simulink model "liftsubsystem"  (R2025b)
settings: Solver=daessc  StartTime=0.0  StopTime=15  FixedStep=1e-3  RelTol=1e-3
values from neighbouring files (symbols this model uses):
  b0 = 1.0    (= 1)    [get_arm_model_with_disturbance.m]    (also in robotParams.m = 3.125)
  beta1 = 3 * omega_o    (= 120)    [robotParams.m]
  beta2 = 3 * omega_o^2    (= 4800)    [robotParams.m]
  beta3 = omega_o^3    (= 64000)    [robotParams.m]
  g = 9.81    [get_arm_model.m]    (also in robotParams.m)
  g_fork = 2*pi*50    (= 314.159265359)    [robotParams.m]
  g_lift = 2*pi*50    (= 314.159265359)    [robotParams.m]
  Kd_fork = 5    [robotParams.m]
  Kd_lift = 5    [robotParams.m]
  Kp_fork = 20    [robotParams.m]
  Kp_lift = 20    [robotParams.m]
  lx = 0.3    [robotParams.m]
  ly = 0.8    [robotParams.m]
  lz = 1    [robotParams.m]
  m = 1    [robotParams.m]
  M = reshape([mt1,mt2,mt3],4,4)    [mass_matrix.m]    (also in robotParams.m = 16)
  m_w = 1    [robotParams.m]
  N = 20    [ocp_arm.m]    (also in ocp_arm_disturbances.m; ocp_lift.m)
  T_control = 1e-3    (= 0.001)    [robotParams.m]
undefined symbols (not defined in the file or in its folder): dspblkCoreblockFVToolHelper, gcbh, K_fd, K_fp, M_n44, Mn_33, Mn_44, X, Y, Z
libraries: sm_lib x257, nesl_utility x58, sharedTrackingLibrary x6, slpidlib x4, simulink x4, robotcorelib x1
(part 2 of 8)

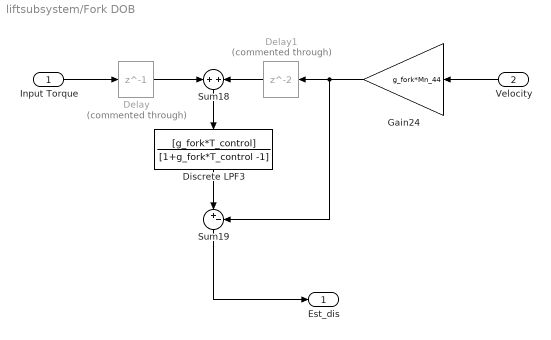
== system liftsubsystem/Fork DOB ==
  Input Torque : Inport
  Velocity : Inport  Port=2
  Delay : Delay  Commented=through  DelayLength=1  InputProcessing=Columns as channels (frame based)  SampleTime=T_control
  Delay1 : Delay  Commented=through  InputProcessing=Columns as channels (frame based)  SampleTime=T_control
  Discrete LPF3 : DiscreteFilter  LoadFcn=dspblkCoreblockFVToolHelper(gcbh,'load');  Numerator=[g_fork*T_control]  Denominator=[1+g_fork*T_control -1]
      settings: CopyFcn=dspblkCoreblockFVToolHelper(gcbh,'copy');  DeleteFcn=dspblkCoreblockFVToolHelper(gcbh,'close');  ModelCloseFcn=dspblkCoreblockFVToolHelper(gcbh,'close');  PreSaveFcn=dspblkCoreblockFVToolHelper(gcbh,'presave');  PostSaveFcn=dspblkCoreblockFVToolHelper(gcbh,'postsave');  CloseFcn=dspblkCoreblockFVToolHelper(gcbh,'close');
  Gain24 : Gain  Gain=g_fork*Mn_44
  Sum18 : Sum  Inputs=+|+
  Sum19 : Sum  Inputs=|+-
  Est_dis : Outport
  wires:
  Delay/1 -> Sum18/1
  Sum19/1 -> Est_dis/1
  Velocity/1 -> Gain24/1
  Input Torque/1 -> Delay/1
  Sum18/1 -> Discrete LPF3/1
  Gain24/1 -> Sum19/2, Delay1/1
  Discrete LPF3/1 -> Sum19/1
  Delay1/1 -> Sum18/2

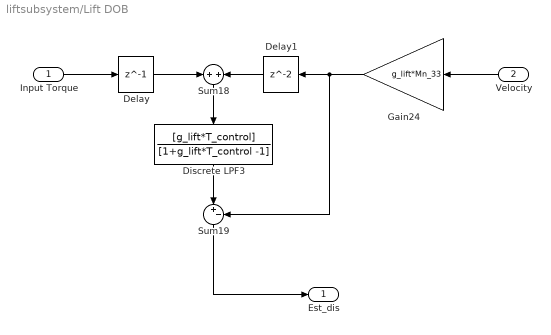
== system liftsubsystem/Lift DOB ==
  Input Torque : Inport
  Velocity : Inport  Port=2
  Delay : Delay  DelayLength=1  InputProcessing=Columns as channels (frame based)  SampleTime=T_control
  Delay1 : Delay  InputProcessing=Columns as channels (frame based)  SampleTime=T_control
  Discrete LPF3 : DiscreteFilter  LoadFcn=dspblkCoreblockFVToolHelper(gcbh,'load');  Numerator=[g_lift*T_control]  Denominator=[1+g_lift*T_control -1]
      settings: CopyFcn=dspblkCoreblockFVToolHelper(gcbh,'copy');  DeleteFcn=dspblkCoreblockFVToolHelper(gcbh,'close');  ModelCloseFcn=dspblkCoreblockFVToolHelper(gcbh,'close');  PreSaveFcn=dspblkCoreblockFVToolHelper(gcbh,'presave');  PostSaveFcn=dspblkCoreblockFVToolHelper(gcbh,'postsave');  CloseFcn=dspblkCoreblockFVToolHelper(gcbh,'close');
  Gain24 : Gain  Gain=g_lift*Mn_33
  Sum18 : Sum  Inputs=+|+
  Sum19 : Sum  Inputs=|+-
  Est_dis : Outport
  wires:
  Delay1/1 -> Sum18/2
  Discrete LPF3/1 -> Sum19/1
  Gain24/1 -> Delay1/1, Sum19/2
  Sum18/1 -> Discrete LPF3/1
  Input Torque/1 -> Delay/1
  Velocity/1 -> Gain24/1
  Sum19/1 -> Est_dis/1
  Delay/1 -> Sum18/1

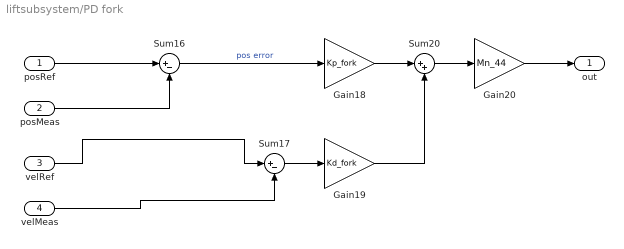
== system liftsubsystem/PD fork ==
  posRef : Inport
  posMeas : Inport  Port=2
  velRef : Inport  Port=3
  velMeas : Inport  Port=4
  Gain18 : Gain  Gain=Kp_fork
  Gain19 : Gain  Gain=Kd_fork
  Gain20 : Gain  Gain=Mn_44
  Sum16 : Sum  Inputs=|+-
  Sum17 : Sum  Inputs=|+-
  Sum20 : Sum  Inputs=|++
  out : Outport
  wires:
  Sum16/1 -> Gain18/1  "pos error"
  Gain18/1 -> Sum20/1
  Sum17/1 -> Gain19/1
  posRef/1 -> Sum16/1
  Sum20/1 -> Gain20/1
  Gain19/1 -> Sum20/2
  Gain20/1 -> out/1
  posMeas/1 -> Sum16/2
  velRef/1 -> Sum17/1
  velMeas/1 -> Sum17/2

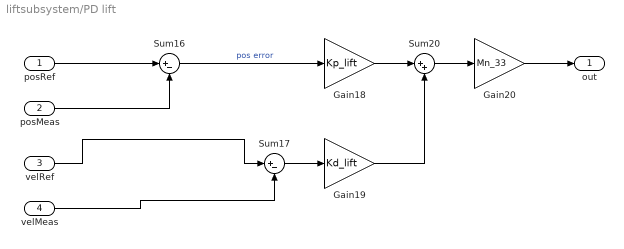
== system liftsubsystem/PD lift ==
  posRef : Inport
  posMeas : Inport  Port=2
  velRef : Inport  Port=3
  velMeas : Inport  Port=4
  Gain18 : Gain  Gain=Kp_lift
  Gain19 : Gain  Gain=Kd_lift
  Gain20 : Gain  Gain=Mn_33
  Sum16 : Sum  Inputs=|+-
  Sum17 : Sum  Inputs=|+-
  Sum20 : Sum  Inputs=|++
  out : Outport
  wires:
  velMeas/1 -> Sum17/2
  velRef/1 -> Sum17/1
  posMeas/1 -> Sum16/2
  Gain20/1 -> out/1
  Gain19/1 -> Sum20/2
  Sum20/1 -> Gain20/1
  posRef/1 -> Sum16/1
  Sum17/1 -> Gain19/1
  Gain18/1 -> Sum20/1
  Sum16/1 -> Gain18/1  "pos error"
